simulink model "JYC"  (R2022b)
settings: Solver=VariableStepAuto  StartTime=0.0  StopTime=10.0  RelTol=1e-3
libraries: spsDiodeLib x4, spsIGBTLib x4, spsACVoltageSourceLib x1, spsSeriesRLCBranchLib x1, spsVoltageMeasurementLib x1
settings Model: Creator=HP  LastModifiedBy=HP

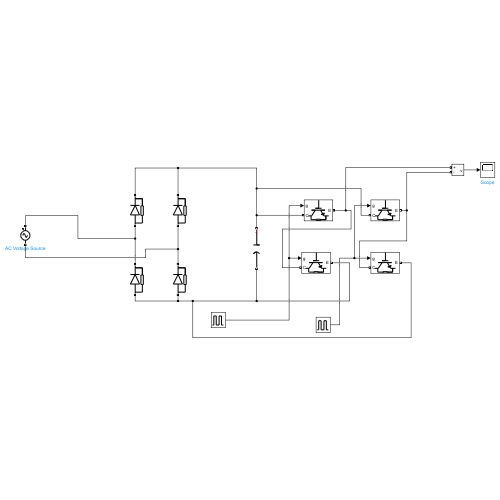
[thumbnail: Simulink's stored preview of the top-level diagram]
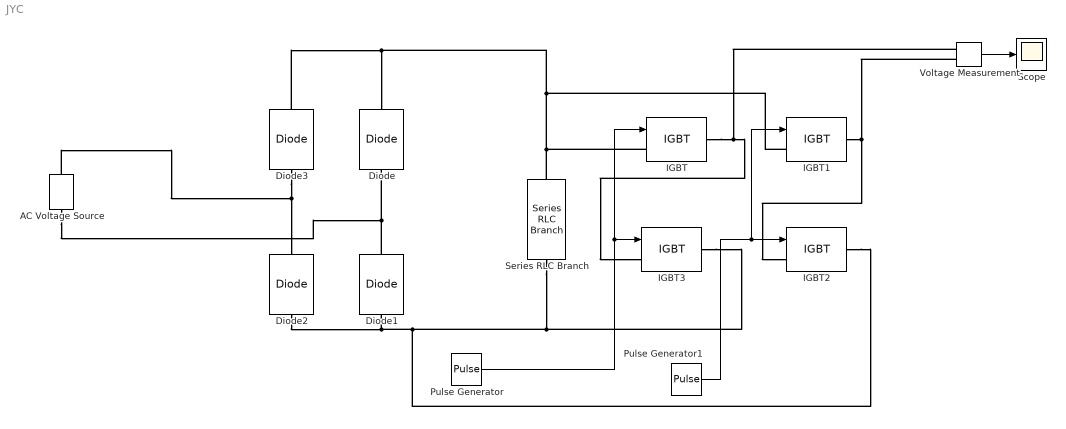
== system JYC ==
  AC Voltage Source : spsACVoltageSourceLib/AC Voltage Source  Amplitude=100  Phase=0  Frequency=60  SampleTime=0  Measurements=None  BusType=swing  Pref=10e3  Qref=0  Qmin=-inf  Qmax=+inf
  Diode{,1..3} (4 alike) : spsDiodeLib/Diode  Ron=0.001  Lon=0  Vf=0.8  IC=0  UseSnubber=0  Rs=500  Cs=250e-9  Measurements=off
  IGBT{,1..3} (4 alike) : spsIGBTLib/IGBT  Ron=0.001  Lon=0  Vf=1  Tf=1e-6  Tt=2e-6  IC=0  Rs=1e5  Cs=inf  Measurements=off
  Pulse Generator : DiscretePulseGenerator  PulseType=Time based  Period=10  PulseWidth=5
  Pulse Generator1 : DiscretePulseGenerator  PulseType=Time based  Period=10  PulseWidth=5
  Scope : Scope
  Series RLC Branch : spsSeriesRLCBranchLib/Series RLC Branch  LConnTagsString=__new0  RConnTagsString=__new0  BranchType=C  Resistance=1  Inductance=1e-3  SetiL0=off  InitialCurrent=0  Capacitance=1e-6  Setx0=off  InitialVoltage=0  Measurements=None
  Voltage Measurement : spsVoltageMeasurementLib/Voltage Measurement  PhasorSimulation=off  OutputType=Complex  PSBequivalent=0
  wires:
  Pulse Generator/1 -> IGBT3/1, IGBT/1
  Pulse Generator1/1 -> IGBT1/1, IGBT2/1
  Voltage Measurement/1 -> Scope/1
  connections:
  Diode3/LConn1 -- AC Voltage Source/RConn1 -- Diode2/RConn1
  Diode1/RConn1 -- AC Voltage Source/LConn1 -- Diode/LConn1
  Diode3/RConn1 -- IGBT1/LConn1 -- Series RLC Branch/LConn1 -- IGBT/LConn1 -- Diode/RConn1
  Diode2/LConn1 -- IGBT3/RConn1 -- Series RLC Branch/RConn1 -- IGBT2/RConn1 -- Diode1/LConn1
  IGBT/RConn1 -- Voltage Measurement/LConn1 -- IGBT3/LConn1
  IGBT1/RConn1 -- IGBT2/LConn1 -- Voltage Measurement/LConn2
